simulink model "SAE_Powertrain"  (R2019b)
settings: Solver=ode1  StartTime=0.0  StopTime=inf  FixedStep=0.0002  RelTol=1e-3
PreLoadFcn:
  | vehicle = 'Car'; if ~length(which('cmself')), cmenv; end
  | SAE_Powertrain_bus
InitFcn:
  | vehicle = 'Car'; if ~length(which('cmself')), cmenv; end
  | SAE_Powertrain_bus
model workspace (MAT data in the model file):
  FRONT = [9 11 12 12 12 14 16 18 19 20 20 25 ... (14 elements, 1x14)]
  REAR = [15 15.7 23 25 25 25 25 25 25 25]
libraries: CarMaker4SL x44
(part 2 of 2)

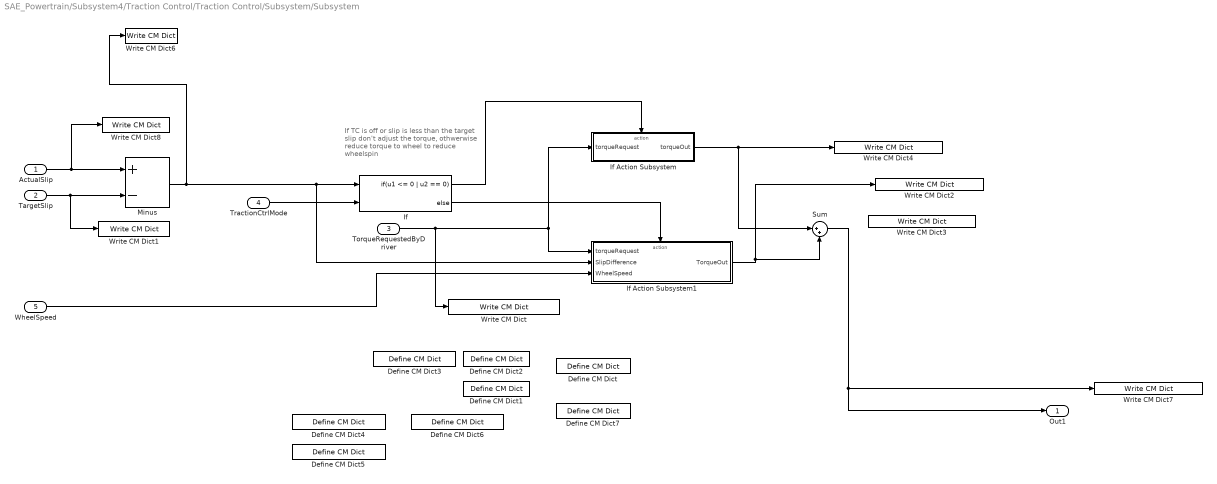
== system SAE_Powertrain/Subsystem4/Traction Control/Traction Control/Subsystem/Subsystem ==
  note: If TC is off or slip is less than the target slip don't adjust the torque,
      | othwerwise reduce torque to wheel to reduce wheelspin
  ActualSlip : Inport
  TargetSlip : Inport  Port=2
  TorqueRequestedByDriver : Inport  Port=3
  TractionCtrlMode : Inport  Port=4
  WheelSpeed : Inport  Port=5
  Define CM Dict : CarMaker4SL/Define CM Dict  xname=Caleb.TorquePidOut  xmono=off  xtype=Double4  xdvaplace=None  xnstates=0  xfirststate=0  xinitial=0
  Define CM Dict1 : CarMaker4SL/Define CM Dict  xname=Caleb.IfOutputTwo  xmono=off  xtype=Double4  xdvaplace=None  xnstates=0  xfirststate=0  xinitial=0
  Define CM Dict2 : CarMaker4SL/Define CM Dict  xname=Caleb.IfOutput  xmono=off  xtype=Double4  xdvaplace=None  xnstates=0  xfirststate=0  xinitial=0
  Define CM Dict3 : CarMaker4SL/Define CM Dict  xname=Caleb.TorqueRequest  xmono=off  xtype=Double4  xdvaplace=None  xnstates=0  xfirststate=0  xinitial=0
  Define CM Dict4 : CarMaker4SL/Define CM Dict  xname=Caleb.TargetSlip  xmono=off  xtype=Double4  xdvaplace=None  xnstates=0  xfirststate=0  xinitial=0
  Define CM Dict5 : CarMaker4SL/Define CM Dict  xname=Caleb.ActualSlip  xmono=off  xtype=Double4  xdvaplace=None  xnstates=0  xfirststate=0  xinitial=0
  Define CM Dict6 : CarMaker4SL/Define CM Dict  xname=Caleb.DiffSlip  xmono=off  xtype=Double4  xdvaplace=None  xnstates=0  xfirststate=0  xinitial=0
  Define CM Dict7 : CarMaker4SL/Define CM Dict  xname=Caleb.TorqueOut  xmono=off  xtype=Double4  xdvaplace=None  xnstates=0  xfirststate=0  xinitial=0
  If : If  NumInputs=2  IfExpression=u1 <= 0 | u2 == 0
  If Action Subsystem : Subsystem  TreatAsAtomicUnit=on
  If Action Subsystem1 : Subsystem  TreatAsAtomicUnit=on
  Minus : Sum  Inputs=+-
  Sum : Sum  Inputs=|++
  Write CM Dict : CarMaker4SL/Write CM Dict  xname=Caleb.TorqueRequest  xsync=off
  Write CM Dict1 : CarMaker4SL/Write CM Dict  xname=Caleb.TargetSlip  xsync=off
  Write CM Dict2 : CarMaker4SL/Write CM Dict  xname=Caleb.IfOutput  xsync=off
  Write CM Dict3 : CarMaker4SL/Write CM Dict  xname=Caleb.TorquePidOut  xsync=off
  Write CM Dict4 : CarMaker4SL/Write CM Dict  xname=Caleb.IfOutputTwo  xsync=off
  Write CM Dict6 : CarMaker4SL/Write CM Dict  xname=Caleb.DiffSlip  xsync=off
  Write CM Dict7 : CarMaker4SL/Write CM Dict  xname=Caleb.TorqueOut  xsync=off
  Write CM Dict8 : CarMaker4SL/Write CM Dict  xname=Caleb.ActualSlip  xsync=off
  Out1 : Outport
  wires:
  If Action Subsystem1/1(TorqueOut) -> Sum/2, Write CM Dict2/1
  TorqueRequestedByDriver/1 -> Write CM Dict/1, If Action Subsystem1/1(torqueRequest), If Action Subsystem/1(torqueRequest)
  If/1 -> If Action Subsystem/Action
  If Action Subsystem/1(torqueOut) -> Sum/1, Write CM Dict4/1
  ActualSlip/1 -> Write CM Dict8/1, Minus/1
  Minus/1 -> Write CM Dict6/1, If Action Subsystem1/2(SlipDifference), If/1
  TargetSlip/1 -> Write CM Dict1/1, Minus/2
  If/2 -> If Action Subsystem1/Action
  TractionCtrlMode/1 -> If/2
  WheelSpeed/1 -> If Action Subsystem1/3(WheelSpeed)
  Sum/1 -> Out1/1, Write CM Dict7/1

== system SAE_Powertrain/Subsystem4/Traction Control/Traction Control/Subsystem/Subsystem1 ==
  note: If TC is off or slip is less than the target slip don't adjust the torque,
      | othwerwise reduce torque to wheel to reduce wheelspin
  ActualSlip : Inport
  TargetSlip : Inport  Port=2
  TorqueRequestedByDriver : Inport  Port=3
  TractionCtrlMode : Inport  Port=4
  WheelSpeed : Inport  Port=5
  If : If  NumInputs=2  IfExpression=u1 <= 0 | u2 == 0
  If Action Subsystem : Subsystem  TreatAsAtomicUnit=on
  If Action Subsystem1 : Subsystem  TreatAsAtomicUnit=on
  Minus : Sum  Inputs=+-
  Sum : Sum  Inputs=|++
  Out1 : Outport
  wires:
  TorqueRequestedByDriver/1 -> If Action Subsystem1/1(torqueRequest), If Action Subsystem/1(torqueRequest)
  If/1 -> If Action Subsystem/Action
  ActualSlip/1 -> Minus/1
  Minus/1 -> If Action Subsystem1/2(SlipDifference), If/1
  TargetSlip/1 -> Minus/2
  If/2 -> If Action Subsystem1/Action
  TractionCtrlMode/1 -> If/2
  WheelSpeed/1 -> If Action Subsystem1/3(WheelSpeed)
  If Action Subsystem/1(torqueOut) -> Sum/1
  If Action Subsystem1/1(TorqueOut) -> Sum/2
  Sum/1 -> Out1/1

== system SAE_Powertrain/Subsystem4/Traction Control/Traction Control/Subsystem1/Subsystem1 ==
  note: If TC is off or slip is less than the target slip don't adjust the torque,
      | othwerwise reduce torque to wheel to reduce wheelspin
  ActualSlip : Inport
  TargetSlip : Inport  Port=2
  TorqueRequestedByDriver : Inport  Port=3
  TractionCtrlMode : Inport  Port=4
  WheelSpeed : Inport  Port=5
  If : If  NumInputs=2  IfExpression=u1 <= 0 | u2 == 0
  If Action Subsystem : Subsystem  TreatAsAtomicUnit=on
  If Action Subsystem1 : Subsystem  TreatAsAtomicUnit=on
  Minus : Sum  Inputs=+-
  Sum : Sum  Inputs=|++
  Out1 : Outport
  wires:
  TorqueRequestedByDriver/1 -> If Action Subsystem1/1(torqueRequest), If Action Subsystem/1(torqueRequest)
  If/1 -> If Action Subsystem/Action
  ActualSlip/1 -> Minus/1
  Minus/1 -> If Action Subsystem1/2(SlipDifference), If/1
  TargetSlip/1 -> Minus/2
  If/2 -> If Action Subsystem1/Action
  TractionCtrlMode/1 -> If/2
  WheelSpeed/1 -> If Action Subsystem1/3(WheelSpeed)
  If Action Subsystem/1(torqueOut) -> Sum/1
  Sum/1 -> Out1/1
  If Action Subsystem1/1(TorqueOut) -> Sum/2

== system SAE_Powertrain/Subsystem4/Traction Control/Traction Control/Subsystem1/Subsystem2 ==
  note: If TC is off or slip is less than the target slip don't adjust the torque,
      | othwerwise reduce torque to wheel to reduce wheelspin
  ActualSlip : Inport
  TargetSlip : Inport  Port=2
  TorqueRequestedByDriver : Inport  Port=3
  TractionCtrlMode : Inport  Port=4
  WheelSpeed : Inport  Port=5
  If : If  NumInputs=2  IfExpression=u1 <= 0 | u2 == 0
  If Action Subsystem : Subsystem  TreatAsAtomicUnit=on
  If Action Subsystem1 : Subsystem  TreatAsAtomicUnit=on
  Minus : Sum  Inputs=+-
  Sum : Sum  Inputs=|++
  Out1 : Outport
  wires:
  TorqueRequestedByDriver/1 -> If Action Subsystem1/1(torqueRequest), If Action Subsystem/1(torqueRequest)
  If/1 -> If Action Subsystem/Action
  ActualSlip/1 -> Minus/1
  Minus/1 -> If Action Subsystem1/2(SlipDifference), If/1
  TargetSlip/1 -> Minus/2
  If/2 -> If Action Subsystem1/Action
  TractionCtrlMode/1 -> If/2
  WheelSpeed/1 -> If Action Subsystem1/3(WheelSpeed)
  Sum/1 -> Out1/1
  If Action Subsystem/1(torqueOut) -> Sum/1
  If Action Subsystem1/1(TorqueOut) -> Sum/2

== system SAE_Powertrain/Subsystem4/Traction Control/Traction Control/Subsystem/Subsystem/If Action Subsystem ==
  torqueRequest : Inport
  Action Port : ActionPort  ActionPortLabel=if(u1 <= 0 | u2 == 0)
  torqueOut : Outport
  wires:
  torqueRequest/1 -> torqueOut/1

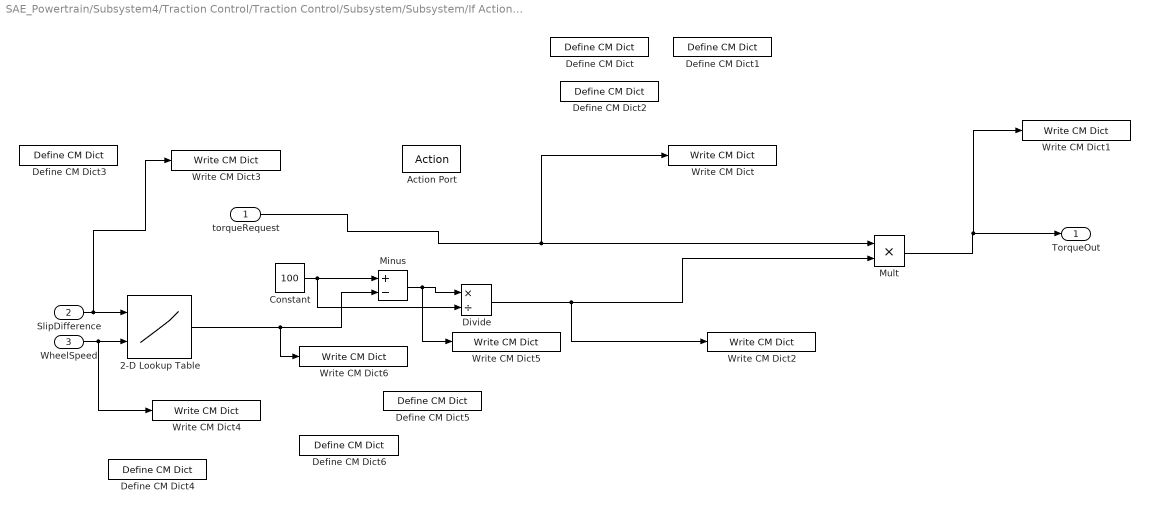
== system SAE_Powertrain/Subsystem4/Traction Control/Traction Control/Subsystem/Subsystem/If Action Subsystem1 ==
  torqueRequest : Inport
  SlipDifference : Inport  Port=2
  WheelSpeed : Inport  Port=3
  Action Port : ActionPort  ActionPortLabel=else
  2-D Lookup Table : Lookup_n-D  BreakpointsForDimension1=[0 0.05 0.1 0.15 0.5 2.5, 15, 35, 50, 100]  BreakpointsForDimension2=[0 500 1000 1500 2000]  Table=[0 0 0 0 0;2 2 2 2 2; 5 5 5 5 5; 7 7 7 7 7; 12 12 12 12 12; 50 50 50 50 50; 50 50 50 50 50; 50 50 50 50 50; 50 50 50 50 50; 50 50 50 50 50]  InternalRulePriority=Speed  RndMeth=Simplest  InputSameDT=on
  Constant : Constant  Value=100
  Define CM Dict : CarMaker4SL/Define CM Dict  xname=Debug.TorqueR  xmono=off  xtype=Double4  xdvaplace=None  xnstates=0  xfirststate=0  xinitial=0
  Define CM Dict1 : CarMaker4SL/Define CM Dict  xname=Debug.TorqueA  xmono=off  xtype=Double4  xdvaplace=None  xnstates=0  xfirststate=0  xinitial=0
  Define CM Dict2 : CarMaker4SL/Define CM Dict  xname=Debug.Table  xmono=off  xtype=Double4  xdvaplace=None  xnstates=0  xfirststate=0  xinitial=0
  Define CM Dict3 : CarMaker4SL/Define CM Dict  xname=Debug.SlipDiff  xmono=off  xtype=Double4  xdvaplace=None  xnstates=0  xfirststate=0  xinitial=0
  Define CM Dict4 : CarMaker4SL/Define CM Dict  xname=Debug.WhlSpeed  xmono=off  xtype=Double4  xdvaplace=None  xnstates=0  xfirststate=0  xinitial=0
  Define CM Dict5 : CarMaker4SL/Define CM Dict  xname=Debug.Percent  xmono=off  xtype=Double4  xdvaplace=None  xnstates=0  xfirststate=0  xinitial=0
  Define CM Dict6 : CarMaker4SL/Define CM Dict  xname=Debug.RawTable  xmono=off  xtype=Double4  xdvaplace=None  xnstates=0  xfirststate=0  xinitial=0
  Divide : Product  Inputs=*/
  Minus : Sum  Inputs=+-
  Mult : Product  Inputs=**
  Write CM Dict : CarMaker4SL/Write CM Dict  xname=Debug.TorqueR  xsync=off
  Write CM Dict1 : CarMaker4SL/Write CM Dict  xname=Debug.TorqueA  xsync=off
  Write CM Dict2 : CarMaker4SL/Write CM Dict  xname=Debug.Table  xsync=off
  Write CM Dict3 : CarMaker4SL/Write CM Dict  xname=Debug.SlipDiff  xsync=off
  Write CM Dict4 : CarMaker4SL/Write CM Dict  xname=Debug.WhlSpeed  xsync=off
  Write CM Dict5 : CarMaker4SL/Write CM Dict  xname=Debug.Percent  xsync=off
  Write CM Dict6 : CarMaker4SL/Write CM Dict  xname=Debug.RawTable  xsync=off
  TorqueOut : Outport
  wires:
  torqueRequest/1 -> Write CM Dict/1, Mult/1
  Mult/1 -> Write CM Dict1/1, TorqueOut/1
  SlipDifference/1 -> Write CM Dict3/1, 2-D Lookup Table/1
  WheelSpeed/1 -> Write CM Dict4/1, 2-D Lookup Table/2
  Constant/1 -> Divide/2, Minus/1
  2-D Lookup Table/1 -> Write CM Dict6/1, Minus/2
  Minus/1 -> Write CM Dict5/1, Divide/1
  Divide/1 -> Write CM Dict2/1, Mult/2

== system SAE_Powertrain/Subsystem4/Traction Control/Traction Control/Subsystem/Subsystem1/If Action Subsystem ==
  torqueRequest : Inport
  Action Port : ActionPort  ActionPortLabel=if(u1 <= 0 | u2 == 0)
  torqueOut : Outport
  wires:
  torqueRequest/1 -> torqueOut/1

== system SAE_Powertrain/Subsystem4/Traction Control/Traction Control/Subsystem/Subsystem1/If Action Subsystem1 ==
  torqueRequest : Inport
  SlipDifference : Inport  Port=2
  WheelSpeed : Inport  Port=3
  Action Port : ActionPort  ActionPortLabel=else
  2-D Lookup Table : Lookup_n-D  BreakpointsForDimension1=[0 0.05 0.1 0.15 0.5 2.5, 15, 35, 50, 100]  BreakpointsForDimension2=[0 500 1000 1500 2000]  Table=[0 0 0 0 0;2 2 2 2 2; 5 5 5 5 5; 7 7 7 7 7; 12 12 12 12 12; 50 50 50 50 50; 50 50 50 50 50; 50 50 50 50 50; 50 50 50 50 50; 50 50 50 50 50]  InternalRulePriority=Speed  RndMeth=Simplest  InputSameDT=on
  Constant : Constant  Value=100
  Divide : Product  Inputs=*/
  Minus : Sum  Inputs=+-
  Mult : Product  Inputs=**
  TorqueOut : Outport
  wires:
  torqueRequest/1 -> Mult/1
  Mult/1 -> TorqueOut/1
  SlipDifference/1 -> 2-D Lookup Table/1
  WheelSpeed/1 -> 2-D Lookup Table/2
  Constant/1 -> Divide/2, Minus/1
  2-D Lookup Table/1 -> Minus/2
  Minus/1 -> Divide/1
  Divide/1 -> Mult/2

== system SAE_Powertrain/Subsystem4/Traction Control/Traction Control/Subsystem1/Subsystem1/If Action Subsystem ==
  torqueRequest : Inport
  Action Port : ActionPort  ActionPortLabel=if(u1 <= 0 | u2 == 0)
  torqueOut : Outport
  wires:
  torqueRequest/1 -> torqueOut/1

== system SAE_Powertrain/Subsystem4/Traction Control/Traction Control/Subsystem1/Subsystem1/If Action Subsystem1 ==
  torqueRequest : Inport
  SlipDifference : Inport  Port=2
  WheelSpeed : Inport  Port=3
  Action Port : ActionPort  ActionPortLabel=else
  2-D Lookup Table : Lookup_n-D  BreakpointsForDimension1=[0 0.05 0.1 0.15 0.5 2.5, 15, 35, 50, 100]  BreakpointsForDimension2=[0 500 1000 1500 2000]  Table=[0 0 0 0 0;2 2 2 2 2; 5 5 5 5 5; 7 7 7 7 7; 12 12 12 12 12; 50 50 50 50 50; 50 50 50 50 50; 50 50 50 50 50; 50 50 50 50 50; 50 50 50 50 50]  InternalRulePriority=Speed  RndMeth=Simplest  InputSameDT=on
  Constant : Constant  Value=100
  Divide : Product  Inputs=*/
  Minus : Sum  Inputs=+-
  Mult : Product  Inputs=**
  TorqueOut : Outport
  wires:
  torqueRequest/1 -> Mult/1
  Mult/1 -> TorqueOut/1
  SlipDifference/1 -> 2-D Lookup Table/1
  WheelSpeed/1 -> 2-D Lookup Table/2
  Constant/1 -> Divide/2, Minus/1
  2-D Lookup Table/1 -> Minus/2
  Minus/1 -> Divide/1
  Divide/1 -> Mult/2

== system SAE_Powertrain/Subsystem4/Traction Control/Traction Control/Subsystem1/Subsystem2/If Action Subsystem ==
  torqueRequest : Inport
  Action Port : ActionPort  ActionPortLabel=if(u1 <= 0 | u2 == 0)
  torqueOut : Outport
  wires:
  torqueRequest/1 -> torqueOut/1

== system SAE_Powertrain/Subsystem4/Traction Control/Traction Control/Subsystem1/Subsystem2/If Action Subsystem1 ==
  torqueRequest : Inport
  SlipDifference : Inport  Port=2
  WheelSpeed : Inport  Port=3
  Action Port : ActionPort  ActionPortLabel=else
  2-D Lookup Table : Lookup_n-D  BreakpointsForDimension1=[0 0.05 0.1 0.15 0.5 2.5, 15, 35, 50, 100]  BreakpointsForDimension2=[0 500 1000 1500 2000]  Table=[0 0 0 0 0;2 2 2 2 2; 5 5 5 5 5; 7 7 7 7 7; 12 12 12 12 12; 50 50 50 50 50; 50 50 50 50 50; 50 50 50 50 50; 50 50 50 50 50; 50 50 50 50 50]  InternalRulePriority=Speed  RndMeth=Simplest  InputSameDT=on
  Constant : Constant  Value=100
  Divide : Product  Inputs=*/
  Minus : Sum  Inputs=+-
  Mult : Product  Inputs=**
  TorqueOut : Outport
  wires:
  torqueRequest/1 -> Mult/1
  Mult/1 -> TorqueOut/1
  SlipDifference/1 -> 2-D Lookup Table/1
  WheelSpeed/1 -> 2-D Lookup Table/2
  Constant/1 -> Divide/2, Minus/1
  2-D Lookup Table/1 -> Minus/2
  Minus/1 -> Divide/1
  Divide/1 -> Mult/2
